simulink model "System_model_discrete_static"  (R2022a)
settings: Solver=FixedStepDiscrete  StartTime=0.0  StopTime=T_final  FixedStep=T_sample  RelTol=1e-3
values from neighbouring files (symbols this model uses):
  A_bar_d = [0.99058344787 -0.000125476588979 -1.03572369058e-05 -0.000112840130565 -4.9197018367e-06 -1.67662830632 -0.0228026014464 -0.00188074381714 -0.019999276241 -0.0008715203213 -0.00015214348792 0.987594206485 ... (100 elements, 10x10)]    [A_bar_d.mat]
  B_bar_d = [0.00129291786986 -6.71376007658e-08 -5.54322132914e-09 -6.10354899312e-08 -2.66151497743e-09 0.269747891814 -1.80552874589e-05 -1.49023321753e-06 -1.61887101691e-05 -7.05777435188e-07 -6.71376007665e-08 0.00108984615129 ... (190 elements, 10x19)]    [B_bar_d.mat]
  BDD_thresh = 0.05    [plot_perform_vs_iter.m]    (also in plot_perform_vs_num_attacks.m; run_model.m = 0.03176)
  C_obsv_d = [0 0 0 0 0 -18.3910466782 17.2834976586 0.26596429707 7.1412513587 0.0956721531682 0.757058744511 -7.14197878204 ... (190 elements, 19x10)]    [C_obsv_d.mat]
  D_obsv_d = [0 0 0 0 0 0 0 0 0 0 0 0 ... (361 elements, 19x19)]    [D_obsv_d.mat]
  I = Ic +mc*d^2+2*mw*L^2+2*Im    (= 0.26903125)    [Run_this_file_for_DDWMR_model.m]    (also in run_model.m = [1;2;9;11;12;16;17]; run_model_for_perform_vs_num_attack.m = sort(randperm(n_meas,n_attack)).'; test_different_horizon_size.m = sort(randperm(n_meas,n_attack)).')
  l = n_meas    (= 19)    [run_model.m]
  L_obsv = place(A_bar_d.',C_obsv_d.',P).'    [run_model.m]
  load_buses = [zeros(n_gen,1); ones(n_bus-n_gen,1)]    [run_model.m]
  max_iter = 1000    [MHFDIA_Basics.m]    (also in Perform_vs_iter.m = Max_iter(idx); run_model.m = 2000; run_model_for_perform_vs_num_attack.m = 300)
  n = 5    [MHFDIA_Basics.m]    (also in discretize_linear_model.m = size(A,1); run_model.m = 10)
  n_bus = 14    [run_model.m]
  n_gen = 5    [run_model.m]
  n_states = 2*n_gen    (= 10)    [run_model.m]
  T = floor(n_x/m)    [MHFDIA_Basics.m]    (also in plot_for_different_horizon_size.m = 20; plot_perform_vs_iter.m = 20; run_model.m = round(2*n))
  T_start_attack = .2*T_final    (= 1.6)    [run_model.m]
  U0 = zeros(m,T)    [run_model.m]
  x0 = zeros(n_states,1)    [run_model.m]
  Y0 = zeros(m,T)    [run_model.m]
undefined symbols (not defined in the file or in its folder): G_T, HT, PhiT, sigbuilder_block, T_start_opt, Theta_T
libraries: simulink x4
settings Model: Creator=oanubi  LastModifiedBy=Abely
settings SolverCC: AlgebraicLoopSolver=TrustRegion
settings DebuggingCC: UnconnectedInputMsg=warning  UnconnectedOutputMsg=warning  UnconnectedLineMsg=warning  SFMachineParentedDataDiag=warning
settings RTWCC: DLArmComputeVersion=19.05

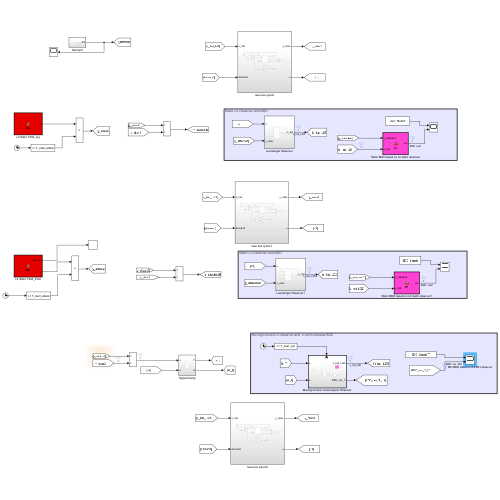
[thumbnail: Simulink's stored preview of the top-level diagram]
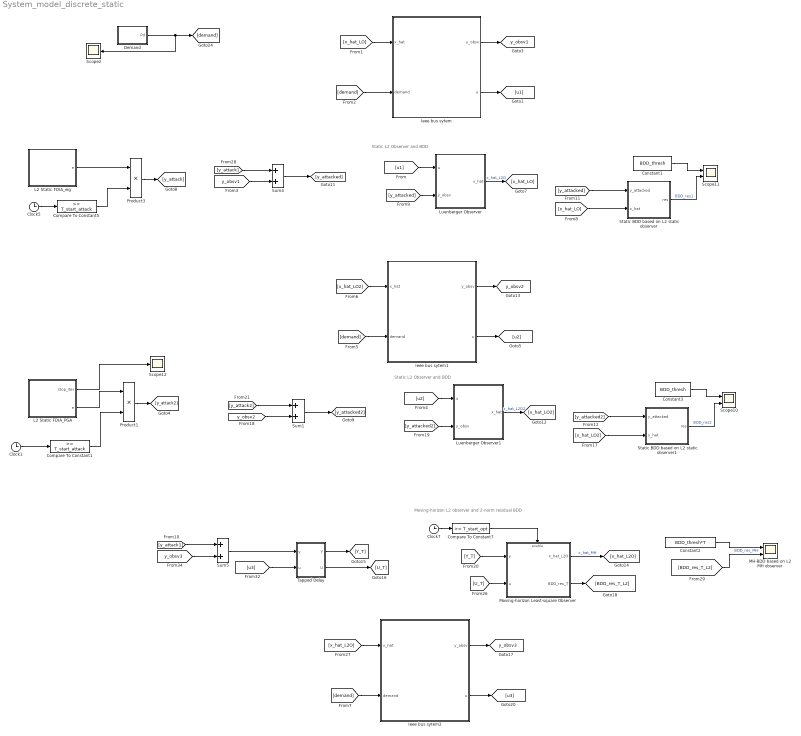
== system System_model_discrete_static ==
  note: Static L2 Observer and BDD
  note: Static L2 Observer and BDD
  note: Moving-horizon L2 observer and 2-norm residual BDD
  Clock1 : Clock
  Clock5 : Clock
  Clock7 : Clock
  Compare To Constant1 : simulink/Logic and Bit Operations/Compare To Constant  relop=>=  const=T_start_attack  OutDataTypeStr=boolean
  Compare To Constant5 : simulink/Logic and Bit Operations/Compare To Constant  relop=>=  const=T_start_attack  OutDataTypeStr=boolean
  Compare To Constant7 : simulink/Logic and Bit Operations/Compare To Constant  relop=>=  const=T_start_opt  OutDataTypeStr=boolean
  Constant1 : Constant  Value=BDD_thresh
  Constant2 : Constant  Value=BDD_thresh*T
  Constant3 : Constant  Value=BDD_thresh
  Demand : Subsystem
  Ieee bus sytem : Subsystem
  Ieee bus sytem1 : Subsystem
  Ieee bus sytem2 : Subsystem
  L2 Static FDIA_PGA : MATLAB Function  TreatAsAtomicUnit=on
  L2 Static FDIA_eig : MATLAB Function  TreatAsAtomicUnit=on
  Luenberger Observer : Subsystem
  Luenberger Observer1 : Subsystem
  MH-BDD based on L2 MH observer : Scope  NumInputPorts=2
  Moving-horizon Least-square Observer : Subsystem
  Product1 : Product
  Product3 : Product
  Scope10 : Scope  NumInputPorts=2
  Scope11 : Scope  NumInputPorts=2
  Scope12 : Scope
  Scope2 : Scope
  Static BDD based on L2 static observer : MATLAB Function  TreatAsAtomicUnit=on
  Static BDD based on L2 static observer1 : MATLAB Function  TreatAsAtomicUnit=on
  Sum1 : Sum
  Sum4 : Sum
  Sum5 : Sum
  Tapped Delay : Subsystem
  tag scope: y_obsv1=global, y_obsv2=global, y_obsv3=global
  wires:
  [y_obsv1] -> Sum4/2
  Sum4/1 -> [y_attacked]
  [y_attack] -> Sum4/1
  [y_attack2] -> Sum1/1
  Sum1/1 -> [y_attacked2]
  [y_obsv2] -> Sum1/2
  Static BDD based on L2 static observer/1(res) -> Scope11/2  "BDD_res1"
  [y_attacked] -> Static BDD based on L2 static observer/1(y_attacked)
  Constant1/1 -> Scope11/1
  [x_hat_LO] -> Static BDD based on L2 static observer/2(x_hat)
  Static BDD based on L2 static observer1/1(res) -> Scope10/2  "BDD_res2"
  Constant3/1 -> Scope10/1
  [y_attacked2] -> Static BDD based on L2 static observer1/1(y_attacked)
  [x_hat_LO2] -> Static BDD based on L2 static observer1/2(x_hat)
  Clock5/1 -> Compare To Constant5/1
  Product3/1 -> [y_attack]
  Compare To Constant5/1 -> Product3/2
  L2 Static FDIA_eig/1(e) -> Product3/1
  L2 Static FDIA_PGA/2(e) -> Product1/1
  Product1/1 -> [y_attack2]
  Compare To Constant1/1 -> Product1/2
  Clock1/1 -> Compare To Constant1/1
  [u1] -> Luenberger Observer/1(u)
  Luenberger Observer/1(x_hat) -> [x_hat_LO]  "x_hat_L2O"
  [y_attacked] -> Luenberger Observer/2(y_obsv)
  [y_attacked2] -> Luenberger Observer1/2(y_obsv)
  [u2] -> Luenberger Observer1/1(u)
  Luenberger Observer1/1(x_hat) -> [x_hat_LO2]  "x_hat_L2O2"
  L2 Static FDIA_PGA/1(stop_iter) -> Scope12/1
  Moving-horizon Least-square Observer/1(x_hat_L2O) -> [x_hat_L2O]  "x_hat_MH"
  [Y_T] -> Moving-horizon Least-square Observer/1(y)
  Compare To Constant7/1 -> Moving-horizon Least-square Observer/Enable
  Constant2/1 -> MH-BDD based on L2 MH observer/1
  Moving-horizon Least-square Observer/2(BDD_res_T) -> [BDD_res_T_L2]
  Clock7/1 -> Compare To Constant7/1
  [U_T] -> Moving-horizon Least-square Observer/2(u)
  [BDD_res_T_L2] -> MH-BDD based on L2 MH observer/2  "BDD_res_MH"
  Sum5/1 -> Tapped Delay/1(y)
  [u3] -> Tapped Delay/2(u)
  Tapped Delay/1(Y) -> [Y_T]
  Tapped Delay/2(U) -> [U_T]
  [x_hat_LO] -> Ieee bus sytem/1(x_hat)
  [demand] -> Ieee bus sytem/2(demand)
  Ieee bus sytem/1(y_obsv) -> [y_obsv1]
  Ieee bus sytem/2(u) -> [u1]
  Demand/1(Pd) -> [demand], Scope2/1
  [demand] -> Ieee bus sytem1/2(demand)
  Ieee bus sytem1/2(u) -> [u2]
  Ieee bus sytem1/1(y_obsv) -> [y_obsv2]
  [x_hat_LO2] -> Ieee bus sytem1/1(x_hat)
  Ieee bus sytem2/1(y_obsv) -> [y_obsv3]
  Ieee bus sytem2/2(u) -> [u3]
  [demand] -> Ieee bus sytem2/2(demand)
  [x_hat_L2O] -> Ieee bus sytem2/1(x_hat)
  [y_obsv3] -> Sum5/2
  [y_attack1] -> Sum5/1

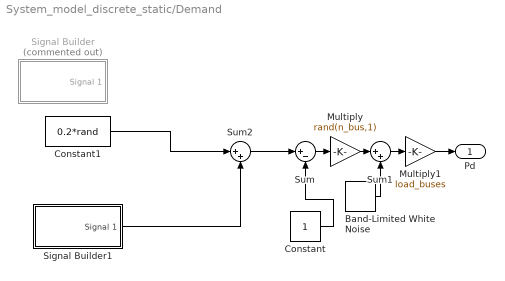
== system System_model_discrete_static/Demand ==
  Band-Limited White Noise : simulink/Sources/Band-Limited White Noise  Cov=1e-8  Ts=0.1  seed=[23341]
  Constant : Constant
  Constant1 : Constant  Value=0.2*rand
  Multiply : Gain  Gain=rand(n_bus,1)
  Multiply1 : Gain  Gain=load_buses
  Signal Builder : Subsystem  Tag=STV Subsys  Commented=on  LoadFcn=sigbuilder_block('load');  StartFcn=sigbuilder_block('start');  StopFcn=sigbuilder_block('stop');  ClipboardFcn=sigbuilder_block('clipboard');  mask(Sigbuilder block){tuvar=[0:10]}
      mask help: Simulink:masks:SigbuilderBlock_MD
      mask init:
      | if ~strcmp(get_param(bdroot(gcbh),'SimulationStatus'),'stopped') tuvar = sigbuilder_block('maskInit'); end
      settings: CopyFcn=sigbuilder_block('copy');  DeleteFcn=sigbuilder_block('delete');  ModelCloseFcn=sigbuilder_block('modelClose');  PreSaveFcn=sigbuilder_block('preSave');  PauseFcn=sigbuilder_block('pause');  ContinueFcn=sigbuilder_block('continue');  NameChangeFcn=sigbuilder_block('namechange');  OpenFcn=sigbuilder_block('open',[439.2 145.2 550.2 399.9 ]);  CloseFcn=sigbuilder_block('close');
      mask Display: plot(0, 0, 100, 100,[2, 2, 32, 32, 2], [68, 8, 8, 68, 68],[32, 2], [38, 38], [32, 19, 2],[53, 60, 44], [32, 17, 17, 2],[16, 16, 31, 31]);txt = getActiveGroup(gcbh);text(2, 100, txt,'verticalAlignment', 'top');
  Signal Builder1 : Subsystem  Tag=STV Subsys  LoadFcn=sigbuilder_block('load');  StartFcn=sigbuilder_block('start');  StopFcn=sigbuilder_block('stop');  ClipboardFcn=sigbuilder_block('clipboard');  mask(Sigbuilder block){tuvar=[0:10]}
      mask help: Simulink:masks:SigbuilderBlock_MD
      mask init:
      | if ~strcmp(get_param(bdroot(gcbh),'SimulationStatus'),'stopped') tuvar = sigbuilder_block('maskInit'); end
      settings: CopyFcn=sigbuilder_block('copy');  DeleteFcn=sigbuilder_block('delete');  ModelCloseFcn=sigbuilder_block('modelClose');  PreSaveFcn=sigbuilder_block('preSave');  PauseFcn=sigbuilder_block('pause');  ContinueFcn=sigbuilder_block('continue');  NameChangeFcn=sigbuilder_block('namechange');  OpenFcn=sigbuilder_block('open',[439.2 145.2 550.2 399.9 ]);  CloseFcn=sigbuilder_block('close');
      mask Display: plot(0, 0, 100, 100,[2, 2, 32, 32, 2], [68, 8, 8, 68, 68],[32, 2], [38, 38], [32, 19, 2],[53, 60, 44], [32, 17, 17, 2],[16, 16, 31, 31]);txt = getActiveGroup(gcbh);text(2, 100, txt,'verticalAlignment', 'top');
  Sum : Sum  Inputs=|+-
  Sum1 : Sum  Inputs=|++
  Sum2 : Sum  Inputs=|++
  Pd : Outport
  wires:
  Sum/1 -> Multiply/1
  Constant/1 -> Sum/2
  Multiply/1 -> Sum1/1
  Band-Limited White Noise/1 -> Sum1/2
  Sum1/1 -> Multiply1/1
  Multiply1/1 -> Pd/1
  Signal Builder1/1(Signal 1) -> Sum2/2
  Constant1/1 -> Sum2/1
  Sum2/1 -> Sum/1

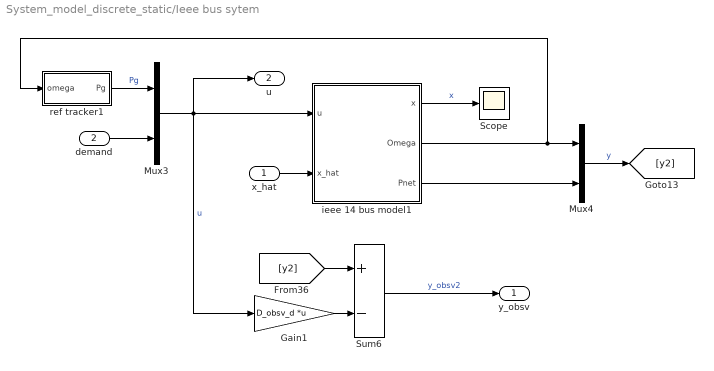
== system System_model_discrete_static/Ieee bus sytem ==
  x_hat : Inport
  demand : Inport  Port=2
  Gain1 : Gain  Gain=D_obsv_d  Multiplication=Matrix(K*u) (u vector)
  Mux3 : Mux  Inputs=2
  Mux4 : Mux  Inputs=2
  Scope : Scope
  Sum6 : Sum  Inputs=+-
  ieee 14 bus model1 : Subsystem
  ref tracker1 : Subsystem
  y_obsv : Outport
  u : Outport  Port=2
  wires:
  demand/1 -> Mux3/2
  Mux4/1 -> [y2]  "y"
  Mux3/1 -> Gain1/1, ieee 14 bus model1/1(u), u/1  "u"
  ref tracker1/1(Pg) -> Mux3/1  "Pg"
  ieee 14 bus model1/1(x) -> Scope/1  "x"
  Gain1/1 -> Sum6/2
  Sum6/1 -> y_obsv/1  "y_obsv2"
  [y2] -> Sum6/1
  ieee 14 bus model1/2(Omega) -> ref tracker1/1(omega), Mux4/1
  x_hat/1 -> ieee 14 bus model1/2(x_hat)
  ieee 14 bus model1/3(Pnet) -> Mux4/2

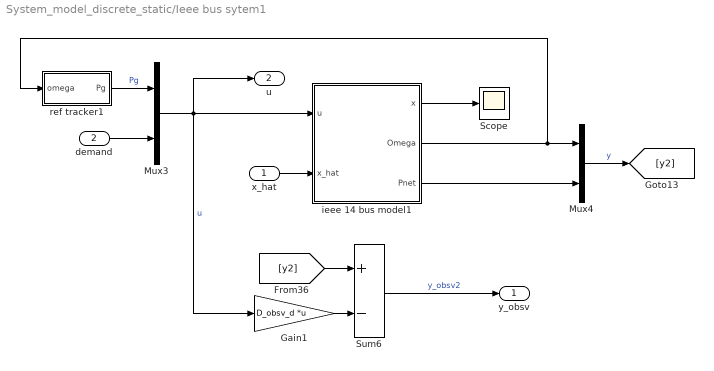
== system System_model_discrete_static/Ieee bus sytem1 ==
  x_hat : Inport
  demand : Inport  Port=2
  Gain1 : Gain  Gain=D_obsv_d  Multiplication=Matrix(K*u) (u vector)
  Mux3 : Mux  Inputs=2
  Mux4 : Mux  Inputs=2
  Scope : Scope
  Sum6 : Sum  Inputs=+-
  ieee 14 bus model1 : Subsystem
  ref tracker1 : Subsystem
  y_obsv : Outport
  u : Outport  Port=2
  wires:
  demand/1 -> Mux3/2
  Mux4/1 -> [y2]  "y"
  Mux3/1 -> Gain1/1, ieee 14 bus model1/1(u), u/1  "u"
  ref tracker1/1(Pg) -> Mux3/1  "Pg"
  ieee 14 bus model1/1(x) -> Scope/1
  Gain1/1 -> Sum6/2
  Sum6/1 -> y_obsv/1  "y_obsv2"
  [y2] -> Sum6/1
  ieee 14 bus model1/2(Omega) -> ref tracker1/1(omega), Mux4/1
  x_hat/1 -> ieee 14 bus model1/2(x_hat)
  ieee 14 bus model1/3(Pnet) -> Mux4/2

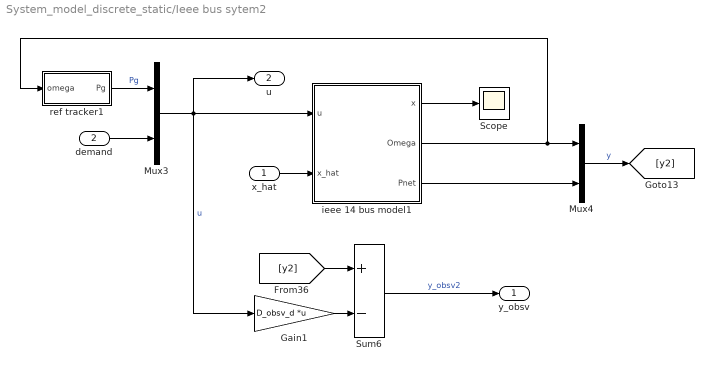
== system System_model_discrete_static/Ieee bus sytem2 ==
  x_hat : Inport
  demand : Inport  Port=2
  Gain1 : Gain  Gain=D_obsv_d  Multiplication=Matrix(K*u) (u vector)
  Mux3 : Mux  Inputs=2
  Mux4 : Mux  Inputs=2
  Scope : Scope
  Sum6 : Sum  Inputs=+-
  ieee 14 bus model1 : Subsystem
  ref tracker1 : Subsystem
  y_obsv : Outport
  u : Outport  Port=2
  wires:
  demand/1 -> Mux3/2
  Mux4/1 -> [y2]  "y"
  Mux3/1 -> Gain1/1, ieee 14 bus model1/1(u), u/1  "u"
  ref tracker1/1(Pg) -> Mux3/1  "Pg"
  ieee 14 bus model1/1(x) -> Scope/1
  Gain1/1 -> Sum6/2
  Sum6/1 -> y_obsv/1  "y_obsv2"
  [y2] -> Sum6/1
  ieee 14 bus model1/2(Omega) -> ref tracker1/1(omega), Mux4/1
  x_hat/1 -> ieee 14 bus model1/2(x_hat)
  ieee 14 bus model1/3(Pnet) -> Mux4/2

== system System_model_discrete_static/Luenberger Observer ==
  u : Inport
  y_obsv : Inport  Port=2
  MATLAB Function : MATLAB Function  TreatAsAtomicUnit=on
  Unit Delay : UnitDelay  InitialCondition=zeros(n_states,1)  SampleTime=-1  HasFrameUpgradeWarning=on
  x_hat : Outport
  wires:
  MATLAB Function/1(x_next) -> Unit Delay/1
  Unit Delay/1 -> x_hat/1, MATLAB Function/1(x)
  u/1 -> MATLAB Function/2(u)
  y_obsv/1 -> MATLAB Function/3(y_obsv)

== system System_model_discrete_static/Luenberger Observer1 ==
  u : Inport
  y_obsv : Inport  Port=2
  MATLAB Function : MATLAB Function  TreatAsAtomicUnit=on
  Unit Delay : UnitDelay  InitialCondition=zeros(n_states,1)  SampleTime=-1  HasFrameUpgradeWarning=on
  x_hat : Outport
  wires:
  MATLAB Function/1(x_next) -> Unit Delay/1
  Unit Delay/1 -> x_hat/1, MATLAB Function/1(x)
  u/1 -> MATLAB Function/2(u)
  y_obsv/1 -> MATLAB Function/3(y_obsv)

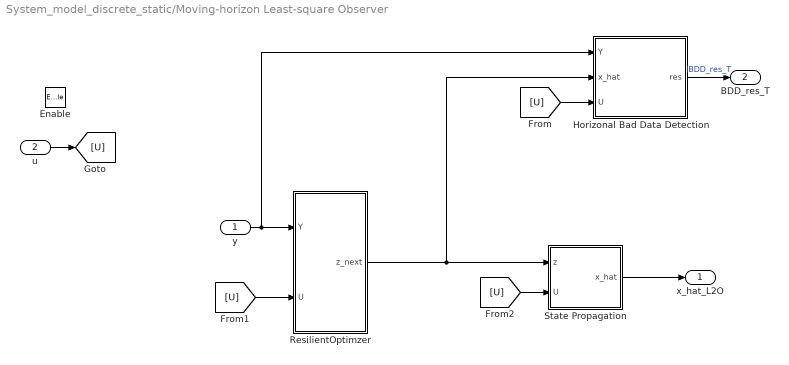
== system System_model_discrete_static/Moving-horizon Least-square Observer ==
  y : Inport
  u : Inport  Port=2
  Enable : EnablePort
  Horizonal Bad Data Detection : MATLAB Function  TreatAsAtomicUnit=on
  ResilientOptimzer : MATLAB Function  TreatAsAtomicUnit=on
  State Propagation : MATLAB Function  TreatAsAtomicUnit=on
  x_hat_L2O : Outport
  BDD_res_T : Outport  Port=2
  wires:
  y/1 -> Horizonal Bad Data Detection/1(Y), ResilientOptimzer/1(Y)
  State Propagation/1(x_hat) -> x_hat_L2O/1
  ResilientOptimzer/1(z_next) -> Horizonal Bad Data Detection/2(x_hat), State Propagation/1(z)
  u/1 -> [U]
  [U] -> Horizonal Bad Data Detection/3(U)
  [U] -> ResilientOptimzer/2(U)
  [U] -> State Propagation/2(U)
  Horizonal Bad Data Detection/1(res) -> BDD_res_T/1  "BDD_res_T"

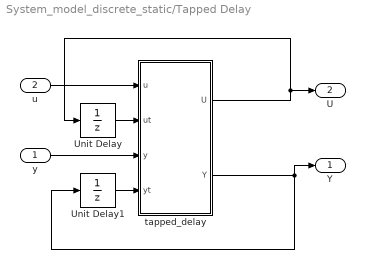
== system System_model_discrete_static/Tapped Delay ==
  y : Inport
  u : Inport  Port=2
  Unit Delay : UnitDelay  InitialCondition=U0  SampleTime=-1  HasFrameUpgradeWarning=on
  Unit Delay1 : UnitDelay  InitialCondition=Y0  SampleTime=-1  HasFrameUpgradeWarning=on
  tapped_delay : MATLAB Function  TreatAsAtomicUnit=on
  Y : Outport
  U : Outport  Port=2
  wires:
  u/1 -> tapped_delay/1(u)
  y/1 -> tapped_delay/3(y)
  tapped_delay/1(U) -> Unit Delay/1, U/1
  tapped_delay/2(Y) -> Y/1, Unit Delay1/1
  Unit Delay/1 -> tapped_delay/2(ut)
  Unit Delay1/1 -> tapped_delay/4(yt)

== system System_model_discrete_static/Demand/Signal Builder ==
  Demux : Demux  Tag=STV Demux  Outputs=1
      settings: DisplayOption=none
  FromWs : FromWorkspace  Tag=STV FromWs  VariableName=tuvar
      SigBuilderData=|
      | common.afterFinalStr = 'Extrapolate'
      | common.sampleTime = 0
      | dataSet.timeRange = [0 10]
      | dataSet.name = 'Group 1'
      | sbobj.Groups.Name = 'Group 1'
      | sbobj.Groups.Signals.Name = 'Signal 1'
      | sbobj.Groups.Signals.XData = [0 0.46 1.5 2.5 4 5 6 7 10]
      | sbobj.Groups.Signals.YData = [1 1.106 1.2 1.2 0.8 0.8 1 1 1]
  Signal 1 : Outport  Tag=STV Outport
  wires:
  Demux/1 -> Signal 1/1
  FromWs/1 -> Demux/1

== system System_model_discrete_static/Demand/Signal Builder1 ==
  Demux : Demux  Tag=STV Demux  Outputs=1
      settings: DisplayOption=none
  FromWs : FromWorkspace  Tag=STV FromWs  VariableName=tuvar
      SigBuilderData=|
      | common.afterFinalStr = 'Extrapolate'
      | common.sampleTime = 0
      | dataSet.timeRange = [0 10]
      | dataSet.name = 'Group 1'
      | sbobj.Groups.Name = 'Group 1'
      | sbobj.Groups.Signals.Name = 'Signal 1'
      | sbobj.Groups.Signals.XData = [0 10]
      | sbobj.Groups.Signals.YData = [0.9 0.9]
  Signal 1 : Outport  Tag=STV Outport
  wires:
  Demux/1 -> Signal 1/1
  FromWs/1 -> Demux/1

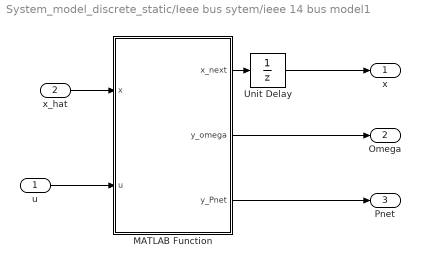
== system System_model_discrete_static/Ieee bus sytem/ieee 14 bus model1 ==
  u : Inport
  x_hat : Inport  Port=2
  MATLAB Function : MATLAB Function  TreatAsAtomicUnit=on
  Unit Delay : UnitDelay  InitialCondition=x0  SampleTime=-1  HasFrameUpgradeWarning=on
  x : Outport
  Omega : Outport  Port=2
  Pnet : Outport  Port=3
  wires:
  MATLAB Function/1(x_next) -> Unit Delay/1
  u/1 -> MATLAB Function/2(u)
  MATLAB Function/2(y_omega) -> Omega/1
  MATLAB Function/3(y_Pnet) -> Pnet/1
  Unit Delay/1 -> x/1
  x_hat/1 -> MATLAB Function/1(x)

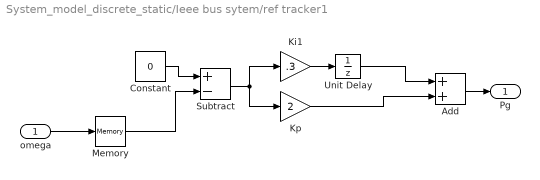
== system System_model_discrete_static/Ieee bus sytem/ref tracker1 ==
  omega : Inport
  Add : Sum
  Constant : Constant  Value=0
  Ki1 : Gain  Gain=.3
  Kp : Gain  Gain=2
  Memory : Memory  InitialCondition=zeros(n_gen,1)
  Subtract : Sum  Inputs=+-
  Unit Delay : UnitDelay  InitialCondition=zeros(n_gen,1)  SampleTime=-1  HasFrameUpgradeWarning=on
  Pg : Outport
  wires:
  Kp/1 -> Add/2
  Unit Delay/1 -> Add/1
  Add/1 -> Pg/1
  Constant/1 -> Subtract/1
  Subtract/1 -> Ki1/1, Kp/1
  Ki1/1 -> Unit Delay/1
  Memory/1 -> Subtract/2
  omega/1 -> Memory/1

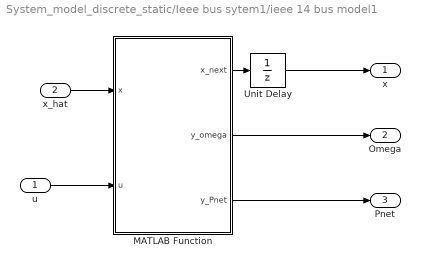
== system System_model_discrete_static/Ieee bus sytem1/ieee 14 bus model1 ==
  u : Inport
  x_hat : Inport  Port=2
  MATLAB Function : MATLAB Function  TreatAsAtomicUnit=on
  Unit Delay : UnitDelay  InitialCondition=x0  SampleTime=-1  HasFrameUpgradeWarning=on
  x : Outport
  Omega : Outport  Port=2
  Pnet : Outport  Port=3
  wires:
  MATLAB Function/1(x_next) -> Unit Delay/1
  u/1 -> MATLAB Function/2(u)
  MATLAB Function/2(y_omega) -> Omega/1
  MATLAB Function/3(y_Pnet) -> Pnet/1
  Unit Delay/1 -> x/1
  x_hat/1 -> MATLAB Function/1(x)

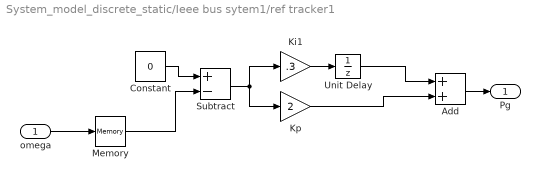
== system System_model_discrete_static/Ieee bus sytem1/ref tracker1 ==
  omega : Inport
  Add : Sum
  Constant : Constant  Value=0
  Ki1 : Gain  Gain=.3
  Kp : Gain  Gain=2
  Memory : Memory  InitialCondition=zeros(n_gen,1)
  Subtract : Sum  Inputs=+-
  Unit Delay : UnitDelay  InitialCondition=zeros(n_gen,1)  SampleTime=-1  HasFrameUpgradeWarning=on
  Pg : Outport
  wires:
  Kp/1 -> Add/2
  Unit Delay/1 -> Add/1
  Add/1 -> Pg/1
  Constant/1 -> Subtract/1
  Subtract/1 -> Ki1/1, Kp/1
  Ki1/1 -> Unit Delay/1
  Memory/1 -> Subtract/2
  omega/1 -> Memory/1

== system System_model_discrete_static/Ieee bus sytem2/ieee 14 bus model1 ==
  u : Inport
  x_hat : Inport  Port=2
  MATLAB Function : MATLAB Function  TreatAsAtomicUnit=on
  Unit Delay : UnitDelay  InitialCondition=x0  SampleTime=-1  HasFrameUpgradeWarning=on
  x : Outport
  Omega : Outport  Port=2
  Pnet : Outport  Port=3
  wires:
  MATLAB Function/1(x_next) -> Unit Delay/1
  u/1 -> MATLAB Function/2(u)
  MATLAB Function/2(y_omega) -> Omega/1
  MATLAB Function/3(y_Pnet) -> Pnet/1
  Unit Delay/1 -> x/1
  x_hat/1 -> MATLAB Function/1(x)

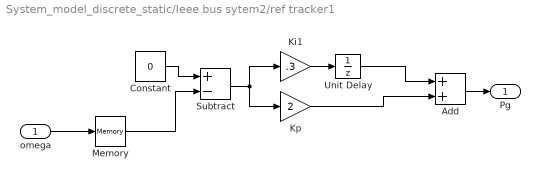
== system System_model_discrete_static/Ieee bus sytem2/ref tracker1 ==
  omega : Inport
  Add : Sum
  Constant : Constant  Value=0
  Ki1 : Gain  Gain=.3
  Kp : Gain  Gain=2
  Memory : Memory  InitialCondition=zeros(n_gen,1)
  Subtract : Sum  Inputs=+-
  Unit Delay : UnitDelay  InitialCondition=zeros(n_gen,1)  SampleTime=-1  HasFrameUpgradeWarning=on
  Pg : Outport
  wires:
  Kp/1 -> Add/2
  Unit Delay/1 -> Add/1
  Add/1 -> Pg/1
  Constant/1 -> Subtract/1
  Subtract/1 -> Ki1/1, Kp/1
  Ki1/1 -> Unit Delay/1
  Memory/1 -> Subtract/2
  omega/1 -> Memory/1

== matlab function System_model_discrete_static/Ieee bus sytem1/ieee 14 bus model1/MATLAB Function ==
  data: x input; x_next output; u input; y_omega output; A_bar_d parameter; C_obsv_d parameter; B_bar_d parameter; D_obsv_d parameter; n_gen parameter; n_bus parameter; y_Pnet output
function [x_next,y_omega,y_Pnet] = fcn(x,u,A_bar_d,C_obsv_d,B_bar_d,D_obsv_d,n_gen, n_bus)
% Discrete state-space model for system

x_next = A_bar_d*x + B_bar_d*u;

y = C_obsv_d*x + D_obsv_d*u;

y_omega = y(1:n_gen);
y_Pnet = y(n_gen+1:n_bus+n_gen);

== matlab function System_model_discrete_static/Tapped Delay/tapped_delay ==
  data: u input; U output; ut input; y input; yt input; Y output
function [U,Y] = fcn(u,ut,y,yt)
%% tapped_delay_array
% shift columns from tapped matrix to the left and appends most recent
% vector to the last column
%%% input
ut(:,1:end-1) = ut(:,2:end);
ut(:,end) = u;
U = ut;
%%% attacked output
yt(:,1:end-1) = yt(:,2:end);
yt(:,end) = y;
Y = yt;

== matlab function System_model_discrete_static/Ieee bus sytem2/ieee 14 bus model1/MATLAB Function ==
  data: x input; x_next output; u input; y_omega output; A_bar_d parameter; C_obsv_d parameter; B_bar_d parameter; D_obsv_d parameter; n_gen parameter; n_bus parameter; y_Pnet output
function [x_next,y_omega,y_Pnet] = fcn(x,u,A_bar_d,C_obsv_d,B_bar_d,D_obsv_d,n_gen, n_bus)
% Discrete state-space model for system

x_next = A_bar_d*x + B_bar_d*u;

y = C_obsv_d*x + D_obsv_d*u;

y_omega = y(1:n_gen);
y_Pnet = y(n_gen+1:n_bus+n_gen);

== matlab function System_model_discrete_static/Moving-horizon Least-square Observer/ResilientOptimzer ==
  data: z_next output; Y input; U input; PhiT parameter; l parameter; T parameter; HT parameter
function z_next  = fcn(Y,U, PhiT,l,T,HT)
u_local = zeros(l,T-1);
u_local(:,:) = U(:,1:end-1);
% vectorized
u = u_local(:);
y = Y(:);

%% estimation
z_next = pinv(PhiT,0.01)*(y-HT*u);

== matlab function System_model_discrete_static/Moving-horizon Least-square Observer/State Propagation ==
  data: z input; U input; x_hat output; Theta_T parameter; n parameter; G_T parameter; T parameter; l parameter
function x_hat = fcn(z,U,Theta_T, n,G_T, T, l)
% x_hat = fcn(z,U,PhiT, HT,n_states)
% Propagates the estimated intial state to the current time
u_local = zeros(l,T-1);
u_local(:,:) = U(:,1:end-1);


% State propagation
x_hat = Theta_T*z(1:n) + G_T*u_local(:);

== matlab function System_model_discrete_static/Moving-horizon Least-square Observer/Horizonal Bad Data Detection ==
  data: Y input; x_hat input; res output; PhiT parameter; HT parameter; l parameter; T parameter; U input
function res = fcn(Y,x_hat,PhiT,HT, l, T, U)
u_local = zeros(l,T-1);
u_local(:,:) = U(:,1:end-1);
% vectorized
u = u_local(:);
y = Y(:);

res = norm(y-PhiT*x_hat-HT*u,2);

== matlab function System_model_discrete_static/L2 Static FDIA_PGA ==
  data: stop_iter output; I parameter; e output; C_obsv_d parameter; BDD_thresh parameter; max_iter parameter
function [stop_iter,e]  = fcn(I,C_obsv_d, BDD_thresh,max_iter)

%% Measurement Channel Attack
%  Assumptions:
%  1. The attacker knows the actual measurement
%  2. The attacker can only corrupt upto n_attack measurements
%  3. The attacker knows the BDD theshold

attack_idx = I;
% e = L2_FDIA(C_obsv_d,attack_idx,0.9*BDD_thresh);

[stop_iter,e] = L2_FDIA2(C_obsv_d,attack_idx,BDD_thresh,max_iter);

== matlab function System_model_discrete_static/Ieee bus sytem/ieee 14 bus model1/MATLAB Function ==
  data: x input; x_next output; u input; y_omega output; A_bar_d parameter; C_obsv_d parameter; B_bar_d parameter; D_obsv_d parameter; n_gen parameter; n_bus parameter; y_Pnet output
function [x_next,y_omega,y_Pnet] = fcn(x,u,A_bar_d,C_obsv_d,B_bar_d,D_obsv_d,n_gen, n_bus)
% Discrete state-space model for system

x_next = A_bar_d*x + B_bar_d*u;

y = C_obsv_d*x + D_obsv_d*u;

y_omega = y(1:n_gen);
y_Pnet = y(n_gen+1:n_bus+n_gen);

== matlab function System_model_discrete_static/Luenberger Observer/MATLAB Function ==
  data: x input; x_next output; u input; y_obsv input; L_obsv parameter; A_bar_d parameter; C_obsv_d parameter; B_bar_d parameter
function x_next  = fcn(x,u,y_obsv,L_obsv,A_bar_d,C_obsv_d,B_bar_d)
% Discrete state-space model for system

x_next = A_bar_d*x + B_bar_d*u + L_obsv*(y_obsv - C_obsv_d*x);

== matlab function System_model_discrete_static/L2 Static FDIA_eig ==
  data: e output; C_obsv_d parameter; BDD_thresh parameter; I parameter
function e = fcn(C_obsv_d, BDD_thresh,I)

%% Measurement Channel Attack
%  Assumptions:
%  1. The attacker knows the actual measurement
%  2. The attacker can only corrupt upto n_attack measurements
%  3. The attacker knows the BDD theshold

attack_idx = I;
e = L2_FDIA(C_obsv_d,attack_idx,BDD_thresh);

== matlab function System_model_discrete_static/Luenberger Observer1/MATLAB Function ==
  data: x input; x_next output; u input; y_obsv input; L_obsv parameter; A_bar_d parameter; C_obsv_d parameter; B_bar_d parameter
function x_next  = fcn(x,u,y_obsv,L_obsv,A_bar_d,C_obsv_d,B_bar_d)
% Discrete state-space model for system

x_next = A_bar_d*x + B_bar_d*u + L_obsv*(y_obsv - C_obsv_d*x);

== matlab function System_model_discrete_static/Static BDD based on L2 static observer1 ==
  data: y_attacked input; x_hat input; res output; C_obsv_d parameter
function res = fcn(y_attacked,x_hat,C_obsv_d)

res = norm(y_attacked-C_obsv_d*x_hat,2);

== matlab function System_model_discrete_static/Static BDD based on L2 static observer ==
  data: y_attacked input; x_hat input; res output; C_obsv_d parameter
function res = fcn(y_attacked,x_hat,C_obsv_d)

res = norm(y_attacked-C_obsv_d*x_hat,2);
